simulink model "NPSS_TTECTrA_sched"  (Simulink 7.5)
settings: Solver=FixedStepDiscrete  StartTime=0.0  StopTime=20  FixedStep=0.02  RelTol=1e-3
undefined symbols (not defined in the file or in its folder): DiscIntNeverNeededParam
libraries: simulink x2
settings Model: Creator=jcsank  LastModifiedBy=jcsank

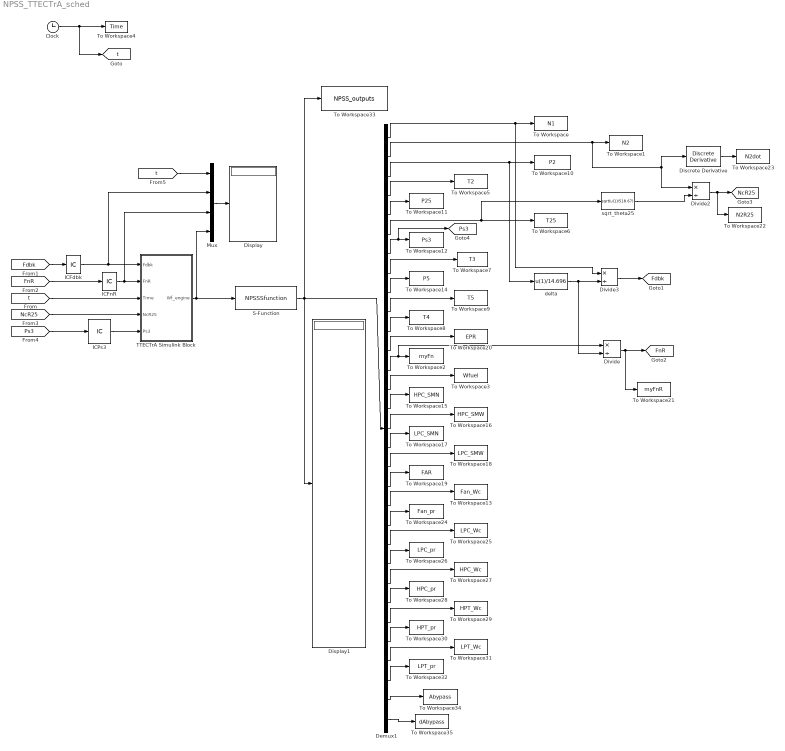
== system NPSS_TTECTrA_sched ==
  Clock : Clock
      settings: Decimation=10
  Demux1 : Demux  Outputs=31
  Discrete Derivative : simulink/Discrete/Discrete Derivative  SystemSampleTime=-1  gainval=1.0  ICPrevScaledInput=0.0  OutMin=[]  OutMax=[]  OutDataType=fixdt(1, 16)  OutScaling=2^-10  DoSatur=off
  Display : Display
  Display1 : Display
  Divide : Product  Inputs=*/
  Divide2 : Product  Inputs=*/
  Divide3 : Product  Inputs=*/
  ICFdbk : InitialCondition  Value=3325.23
  ICFnR : InitialCondition  Value=15000
  ICPs3 : InitialCondition  Value=288.259
  Mux : Mux
  S-Function : S-Function  FunctionName=NPSSSfunction  Parameters='150_PAX_Sfunction.config'  EnableBusSupport=off
  TTECTrA Simulink Block : Subsystem
  To Workspace : ToWorkspace  VariableName=N1  SampleTime=-1  SaveFormat=Array
  To Workspace1 : ToWorkspace  VariableName=N2  SampleTime=-1  SaveFormat=Array
  To Workspace10 : ToWorkspace  VariableName=P2  SampleTime=-1  SaveFormat=Array
  To Workspace11 : ToWorkspace  VariableName=P25  SampleTime=-1  SaveFormat=Array
  To Workspace12 : ToWorkspace  VariableName=Ps3  SampleTime=-1  SaveFormat=Array
  To Workspace13 : ToWorkspace  VariableName=Fan_Wc  SampleTime=-1  SaveFormat=Array
  To Workspace14 : ToWorkspace  VariableName=P5  SampleTime=-1  SaveFormat=Array
  To Workspace15 : ToWorkspace  VariableName=HPC_SMN  SampleTime=-1  SaveFormat=Array
  To Workspace16 : ToWorkspace  VariableName=HPC_SMW  SampleTime=-1  SaveFormat=Array
  To Workspace17 : ToWorkspace  VariableName=LPC_SMN  SampleTime=-1  SaveFormat=Array
  To Workspace18 : ToWorkspace  VariableName=LPC_SMW  SampleTime=-1  SaveFormat=Array
  To Workspace19 : ToWorkspace  VariableName=FAR  SampleTime=-1  SaveFormat=Array
  To Workspace2 : ToWorkspace  VariableName=myFn  SampleTime=-1  SaveFormat=Array
  To Workspace20 : ToWorkspace  VariableName=EPR  SampleTime=-1  SaveFormat=Array
  To Workspace21 : ToWorkspace  VariableName=myFnR  SampleTime=-1  SaveFormat=Array
  To Workspace22 : ToWorkspace  VariableName=N2R25  SampleTime=-1  SaveFormat=Array
  To Workspace23 : ToWorkspace  VariableName=N2dot  SampleTime=-1  SaveFormat=Array
  To Workspace24 : ToWorkspace  VariableName=Fan_pr  SampleTime=-1  SaveFormat=Array
  To Workspace25 : ToWorkspace  VariableName=LPC_Wc  SampleTime=-1  SaveFormat=Array
  To Workspace26 : ToWorkspace  VariableName=LPC_pr  SampleTime=-1  SaveFormat=Array
  To Workspace27 : ToWorkspace  VariableName=HPC_Wc  SampleTime=-1  SaveFormat=Array
  To Workspace28 : ToWorkspace  VariableName=HPC_pr  SampleTime=-1  SaveFormat=Array
  To Workspace29 : ToWorkspace  VariableName=HPT_Wc  SampleTime=-1  SaveFormat=Array
  To Workspace3 : ToWorkspace  VariableName=Wfuel  SampleTime=-1  SaveFormat=Array
  To Workspace30 : ToWorkspace  VariableName=HPT_pr  SampleTime=-1  SaveFormat=Array
  To Workspace31 : ToWorkspace  VariableName=LPT_Wc  SampleTime=-1  SaveFormat=Array
  To Workspace32 : ToWorkspace  VariableName=LPT_pr  SampleTime=-1  SaveFormat=Array
  To Workspace33 : ToWorkspace  VariableName=NPSS_outputs  SampleTime=-1  SaveFormat=Array
  To Workspace34 : ToWorkspace  VariableName=Abypass  SampleTime=-1  SaveFormat=Array
  To Workspace35 : ToWorkspace  VariableName=dAbypass  SampleTime=-1  SaveFormat=Array
  To Workspace4 : ToWorkspace  VariableName=Time  SampleTime=-1  SaveFormat=Array
  To Workspace5 : ToWorkspace  VariableName=T2  SampleTime=-1  SaveFormat=Array
  To Workspace6 : ToWorkspace  VariableName=T25  SampleTime=-1  SaveFormat=Array
  To Workspace7 : ToWorkspace  VariableName=T3  SampleTime=-1  SaveFormat=Array
  To Workspace8 : ToWorkspace  VariableName=T4  SampleTime=-1  SaveFormat=Array
  To Workspace9 : ToWorkspace  VariableName=T5  SampleTime=-1  SaveFormat=Array
  delta : Fcn  Expr=u(1)/14.696
  sqrt_theta25 : Fcn  Expr=sqrt(u(1)/518.67)
  tag scope: Fdbk=global, FnR=global, NcR25=global, Ps3=global, t=global
  wires:
  S-Function/1 -> Demux1/1, Display1/1, To Workspace33/1
  Clock/1 -> [t], To Workspace4/1
  TTECTrA Simulink Block/1(Wf_engine) -> Mux/4, S-Function/1
  [t] -> TTECTrA Simulink Block/3(Time)
  [Fdbk] -> ICFdbk/1
  [FnR] -> ICFnR/1
  [NcR25] -> TTECTrA Simulink Block/4(NcR25)
  Divide/1 -> [FnR], To Workspace21/1
  Divide2/1 -> [NcR25], To Workspace22/1
  Discrete Derivative/1 -> To Workspace23/1
  [t] -> Mux/1
  Mux/1 -> Display/1
  [Ps3] -> ICPs3/1
  Demux1/1 -> To Workspace/1, Divide3/1
  Demux1/2 -> To Workspace1/1, Divide2/1, Discrete Derivative/1
  Demux1/3 -> To Workspace10/1, delta/1
  Demux1/4 -> To Workspace5/1
  Demux1/5 -> To Workspace11/1
  Demux1/6 -> To Workspace6/1, sqrt_theta25/1
  Demux1/7 -> To Workspace12/1, [Ps3]
  Demux1/8 -> To Workspace7/1
  Demux1/10 -> To Workspace9/1
  Demux1/9 -> To Workspace14/1
  Demux1/11 -> To Workspace8/1
  Demux1/12 -> To Workspace20/1
  Demux1/13 -> To Workspace2/1, Divide/1
  Demux1/14 -> To Workspace3/1
  Demux1/15 -> To Workspace15/1
  Demux1/16 -> To Workspace16/1
  Demux1/17 -> To Workspace17/1
  Demux1/18 -> To Workspace18/1
  Demux1/19 -> To Workspace19/1
  sqrt_theta25/1 -> Divide2/2
  Divide3/1 -> [Fdbk]
  ICFdbk/1 -> TTECTrA Simulink Block/1(Fdbk), Mux/2
  ICPs3/1 -> TTECTrA Simulink Block/5(Ps3)
  ICFnR/1 -> TTECTrA Simulink Block/2("FnR "), Mux/3
  delta/1 -> Divide3/2, Divide/2
  Demux1/20 -> To Workspace13/1
  Demux1/21 -> To Workspace24/1
  Demux1/22 -> To Workspace25/1
  Demux1/23 -> To Workspace26/1
  Demux1/24 -> To Workspace27/1
  Demux1/25 -> To Workspace28/1
  Demux1/26 -> To Workspace29/1
  Demux1/27 -> To Workspace30/1
  Demux1/28 -> To Workspace31/1
  Demux1/29 -> To Workspace32/1
  Demux1/30 -> To Workspace34/1
  Demux1/31 -> To Workspace35/1

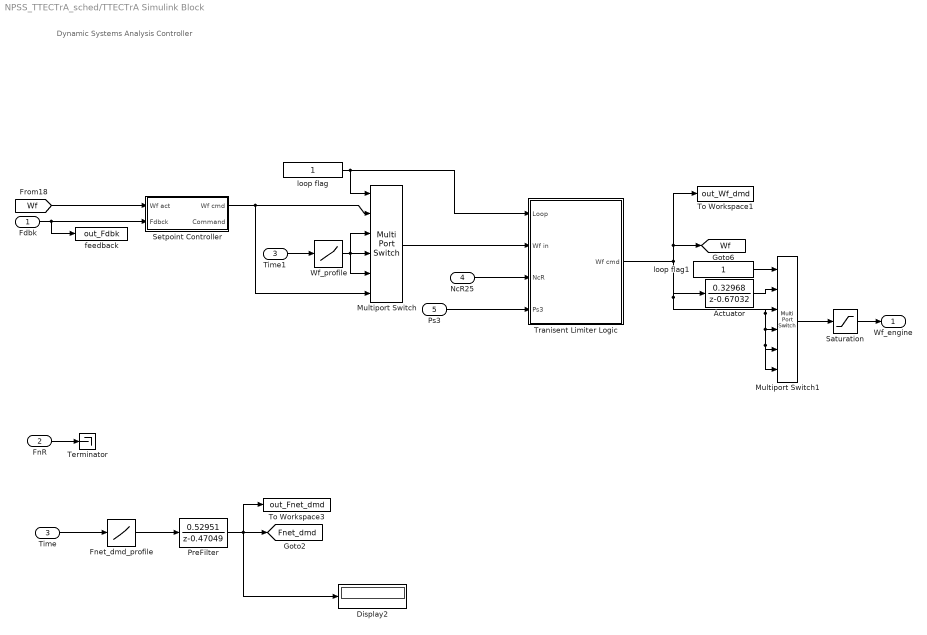
== system NPSS_TTECTrA_sched/TTECTrA Simulink Block ==
  note: Dynamic Systems Analysis Controller
  Fdbk : Inport
  "FnR " : Inport  Port=2
  Time : Inport  Port=3
  NcR25 : Inport  Port=4
  Ps3 : Inport  Port=5
  Actuator : DiscreteTransferFcn  Numerator=[0.32968]  Denominator="[1    -0.67032]"  InitialStates=[0.8029]  SampleTime=-1
  Display2 : Display
  Fnet_dmd_profile : Lookup  InputValues="[0            20            22            34            35            40          40.5            50          50.5            60            95           100]"  Table="[15000  15000  26000  26000  15000  15000  37000  37000  15000  15000  37000  37000]"  SampleTime=0.02
  Multiport Switch : MultiPortSwitch  Inputs=5  zeroidx=off  SampleTime=0.02
  Multiport Switch1 : MultiPortSwitch  Inputs=5  zeroidx=off  SampleTime=0.02
  PreFilter : DiscreteTransferFcn  Numerator=[0.52951]  Denominator="[1    -0.47049]"  InitialStates=[15000]  SampleTime=-1
  Saturation : Saturate  UpperLimit=9999  LowerLimit=0
  Setpoint Controller : Subsystem
  Terminator : Terminator
  Time1 : InportShadow  Port=3
  To Workspace1 : ToWorkspace  VariableName=out_Wf_dmd  SampleTime=-1  SaveFormat=Array
  To Workspace3 : ToWorkspace  VariableName=out_Fnet_dmd  SampleTime=-1  SaveFormat=Array
  Tranisent Limiter Logic : Subsystem
  Wf_profile : Lookup  InputValues="[0            20            22            34            35            40          40.5            50          50.5            60            95           100]"  Table="[0.5         0.5         0.5         0.5         0.5         0.5         0.5         0.5         0.5         0.5         0.5         0.5]"  SampleTime=0.02
  feedback : ToWorkspace  VariableName=out_Fdbk  SampleTime=-1  SaveFormat=Array
  loop flag : Constant
  loop flag1 : Constant
  Wf_engine : Outport
  tag scope: Fnet_dmd=global, Wf=global
  wires:
  [Wf] -> Setpoint Controller/1(Wf act)
  Fdbk/1 -> feedback/1, Setpoint Controller/2(Fdbck)
  Time/1 -> Fnet_dmd_profile/1
  NcR25/1 -> Tranisent Limiter Logic/3(NcR)
  Fnet_dmd_profile/1 -> PreFilter/1
  PreFilter/1 -> [Fnet_dmd], To Workspace3/1, Display2/1
  Saturation/1 -> Wf_engine/1
  Multiport Switch1/1 -> Saturation/1
  loop flag1/1 -> Multiport Switch1/1
  Ps3/1 -> Tranisent Limiter Logic/4(Ps3)
  Time1/1 -> Wf_profile/1
  loop flag/1 -> Tranisent Limiter Logic/1(Loop), Multiport Switch/1
  Multiport Switch/1 -> Tranisent Limiter Logic/2(Wf in)
  Wf_profile/1 -> Multiport Switch/4, Multiport Switch/3, Multiport Switch/5
  Setpoint Controller/1(Wf cmd) -> Multiport Switch/2, Multiport Switch/6
  "FnR "/1 -> Terminator/1
  Actuator/1 -> Multiport Switch1/2
  Tranisent Limiter Logic/1(Wf cmd) -> [Wf], To Workspace1/1, Actuator/1, Multiport Switch1/3, Multiport Switch1/4, Multiport Switch1/5, Multiport Switch1/6

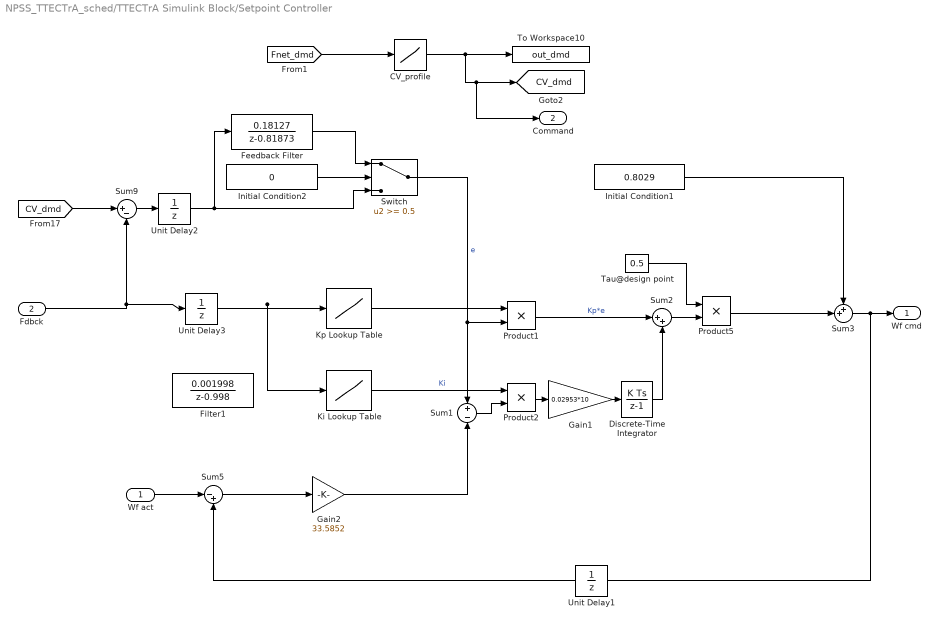
== system NPSS_TTECTrA_sched/TTECTrA Simulink Block/Setpoint Controller ==
  Wf act : Inport
  Fdbck : Inport  Port=2
  CV_profile : Lookup  InputValues="[15000  16100  17200  18300  19400  20500  21600  22700  23800  24900  26000  27100  28200  29300  30400  31500  32600  33700  34800  35900  37000]"  Table="[3325.23        3427.94        3530.34         3632.4        3727.55         3814.4        3903.37        3990.93        4076.84        4162.24        4245.48        4324.93        4403.74        4482.08        4554.24           4626        4697.19        4767.81        4837.69        4908.05        4978.43]"  LookUpMeth=Interpolation-Use End Values  SampleTime=0.02
  Discrete-Time Integrator : DiscreteIntegrator  SampleTime=-1  ICPrevOutput=DiscIntNeverNeededParam  ICPrevScaledInput=DiscIntNeverNeededParam
  Feedback Filter : DiscreteTransferFcn  Numerator=[0.18127]  Denominator="[1    -0.81873]"  SampleTime=0.02
  Filter1 : DiscreteTransferFcn  Numerator=[0.001998]  Denominator="[1      -0.998]"  SampleTime=0.02
  Gain1 : Gain  Gain=0.02953*10
  Gain2 : Gain  Gain=33.5852
  Initial Condition1 : Constant  Value=0.8029
  Initial Condition2 : Constant  Value=0
  Ki Lookup Table : Lookup_n-D  NumberOfTableDimensions=1  BreakpointsForDimension1="[3325.23        3427.94        3530.35        3632.41        3727.55         3814.4        3903.37        3990.93        4076.84        4162.24        4245.48        4324.93        4403.73        4482.08        4554.24           4626        4697.19        4767.81        4837.69        4908.05        4978.43]"  Table="[0.015051    0.015444    0.015341    0.017065    0.020046    0.020556    0.020946    0.022037    0.022631    0.023103    0.024251     0.02523    0.026308    0.028729    0.030476    0.030781    0.032445    0.033214    0.032185    0.032086    0.034071]"  SampleTime=0.02  RndMeth=Simplest  InputSameDT=on
  Kp Lookup Table : Lookup_n-D  NumberOfTableDimensions=1  BreakpointsForDimension1="[3325.23        3427.94        3530.35        3632.41        3727.55         3814.4        3903.37        3990.93        4076.84        4162.24        4245.48        4324.93        4403.73        4482.08        4554.24           4626        4697.19        4767.81        4837.69        4908.05        4978.43]"  Table="[0.0033942   0.0034271   0.0034167   0.0034139   0.0033724   0.0034011   0.0034128   0.0034016   0.0034168   0.0034462   0.0034167   0.0034099   0.0033799   0.0034958   0.0034346   0.0034205   0.0035406    0.003412   0.0037437   0.0037018   0.0038138]"  SampleTime=0.02  RndMeth=Simplest  InputSameDT=on
  Product1 : Product  SampleTime=0.02  RndMeth=Zero
  Product2 : Product  RndMeth=Zero
  Product5 : Product  SampleTime=0.02  RndMeth=Zero
  Sum1 : Sum  Inputs=+|-
  Sum2 : Sum  Inputs=|++  SampleTime=0.02
  Sum3 : Sum  Inputs=++|  SampleTime=0.02
  Sum5 : Sum  Inputs=|-+
  Sum9 : Sum  Inputs=|+-  SampleTime=0.02
  Switch : Switch  Threshold=0.5  SampleTime=0.02
  Tau@design point : Constant  Value=0.5
  To Workspace10 : ToWorkspace  VariableName=out_dmd  SampleTime=-1  SaveFormat=Array
  Unit Delay1 : UnitDelay  SampleTime=-1
  Unit Delay2 : UnitDelay  SampleTime=-1
  Unit Delay3 : UnitDelay  SampleTime=-1
  Wf cmd : Outport
  Command : Outport  Port=2
  tag scope: CV_dmd=global
  wires:
  Tau@design point/1 -> Product5/1
  Product1/1 -> Sum2/1  "Kp*e"
  Product2/1 -> Gain1/1
  Sum9/1 -> Unit Delay2/1
  [CV_dmd] -> Sum9/1
  Wf act/1 -> Sum5/1
  Sum5/1 -> Gain2/1
  Switch/1 -> Product1/2, Sum1/1  "e"
  Sum1/1 -> Product2/2
  Sum2/1 -> Product5/2
  Gain2/1 -> Sum1/2
  Sum3/1 -> Wf cmd/1, Unit Delay1/1
  Initial Condition1/1 -> Sum3/1
  Product5/1 -> Sum3/2
  Gain1/1 -> Discrete-Time Integrator/1
  Discrete-Time Integrator/1 -> Sum2/2
  Ki Lookup Table/1 -> Product2/1  "Ki"
  Fdbck/1 -> Sum9/2, Unit Delay3/1
  CV_profile/1 -> To Workspace10/1, [CV_dmd], Command/1
  [Fnet_dmd] -> CV_profile/1
  Kp Lookup Table/1 -> Product1/1
  Initial Condition2/1 -> Switch/2
  Feedback Filter/1 -> Switch/1
  Unit Delay1/1 -> Sum5/2
  Unit Delay2/1 -> Switch/3, Feedback Filter/1
  Unit Delay3/1 -> Kp Lookup Table/1, Ki Lookup Table/1

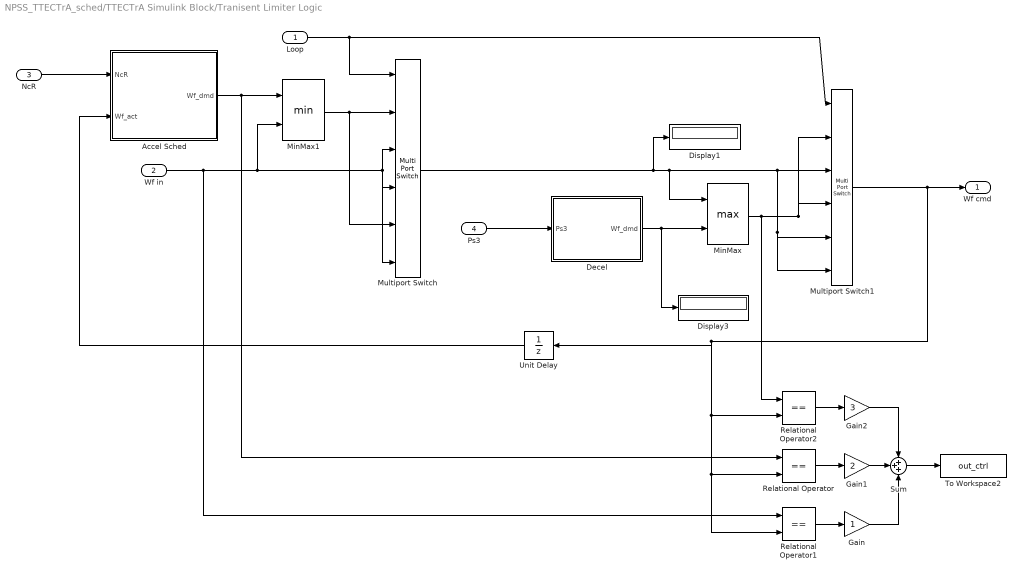
== system NPSS_TTECTrA_sched/TTECTrA Simulink Block/Tranisent Limiter Logic ==
  Loop : Inport
  Wf in : Inport  Port=2
  NcR : Inport  Port=3
  Ps3 : Inport  Port=4
  Accel Sched : Subsystem
  Decel : Subsystem
  Display1 : Display
  Display3 : Display
  Gain : Gain  ParameterDataType=fixdt(1, 16)  ParameterScaling=2^0  OutDataType=fixdt(1, 16)  OutScaling=2^0
  Gain1 : Gain  Gain=2  ParameterDataType=fixdt(1, 16)  ParameterScaling=2^0  OutDataType=fixdt(1, 16)  OutScaling=2^0
  Gain2 : Gain  Gain=3  ParameterDataType=fixdt(1, 16)  ParameterScaling=2^0  OutDataType=fixdt(1, 16)  OutScaling=2^0
  MinMax : MinMax  Function=max  Inputs=2  SampleTime=0.02
  MinMax1 : MinMax  Inputs=2  SampleTime=0.02
  Multiport Switch : MultiPortSwitch  Inputs=5  zeroidx=off  SampleTime=0.02
  Multiport Switch1 : MultiPortSwitch  Inputs=5  zeroidx=off  SampleTime=0.02
  Relational Operator : RelationalOperator  Operator===  LogicOutDataTypeMode=boolean  LogicDataType=fixdt(0, 8)  OutDataTypeStr=boolean
  Relational Operator1 : RelationalOperator  Operator===  LogicOutDataTypeMode=boolean  LogicDataType=fixdt(0, 8)  OutDataTypeStr=boolean
  Relational Operator2 : RelationalOperator  Operator===  LogicOutDataTypeMode=boolean  LogicDataType=fixdt(0, 8)  OutDataTypeStr=boolean
  Sum : Sum  Inputs=+++  OutDataType=fixdt(1, 16)  OutScaling=2^0
  To Workspace2 : ToWorkspace  VariableName=out_ctrl  SampleTime=-1  SaveFormat=Array
  Unit Delay : UnitDelay  SampleTime=-1
  Wf cmd : Outport
  wires:
  NcR/1 -> Accel Sched/1(NcR)
  Unit Delay/1 -> Accel Sched/2(Wf_act)
  Loop/1 -> Multiport Switch/1, Multiport Switch1/1
  Accel Sched/1(Wf_dmd) -> MinMax1/1, Relational Operator/1
  Wf in/1 -> Multiport Switch/3, Multiport Switch/6, Multiport Switch/4, MinMax1/2, Relational Operator1/1
  Ps3/1 -> Decel/1(Ps3)
  Multiport Switch1/1 -> Wf cmd/1, Unit Delay/1, Relational Operator2/2, Relational Operator1/2, Relational Operator/2
  MinMax/1 -> Multiport Switch1/4, Multiport Switch1/2, Relational Operator2/1
  Multiport Switch/1 -> MinMax/1, Multiport Switch1/3, Multiport Switch1/5, Multiport Switch1/6, Display1/1
  Decel/1(Wf_dmd) -> MinMax/2, Display3/1
  MinMax1/1 -> Multiport Switch/2, Multiport Switch/5
  Relational Operator2/1 -> Gain2/1
  Relational Operator/1 -> Gain1/1
  Relational Operator1/1 -> Gain/1
  Gain2/1 -> Sum/1
  Gain1/1 -> Sum/2
  Gain/1 -> Sum/3
  Sum/1 -> To Workspace2/1

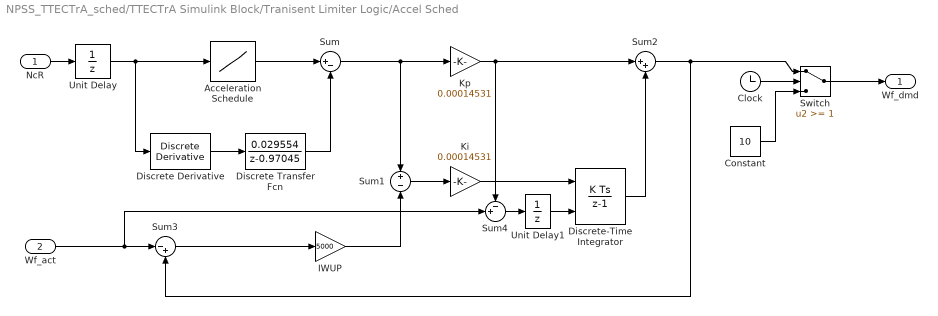
== system NPSS_TTECTrA_sched/TTECTrA Simulink Block/Tranisent Limiter Logic/Accel Sched ==
  NcR : Inport
  Wf_act : Inport  Port=2
  Acceleration Schedule : Lookup  InputValues="[11330  11371  11412  11453  11494  11535  11576  11617  11658  11699  11740  11781  11822  11863  11904  11945  11986  12027  12068  12109  12150  12191  12232  12273  12314  12355  12396  12437  12478  12519  12560  12601  12642  12683  12724  12765  12806  12847  12888  12929  12970]"  Table="[826.80549      826.80549      826.80549      826.80549      826.80549      826.80549      826.80549      826.80549      826.80549      826.80549      826.80549      826.80549      826.80549      826.80549      826.80549       2169.861      4472.7176      5790.6525      6685.5108      7356.4809      7889.4598      8320.7829      8651.7771      8926.4633      9163.2695      9366.3519      9514.0686      9602.0353      9629.1247      9600.4931      9532.9363      9449.8108        9338.03      9159.9036      826.80549      826.80549      826.80549      826.80549      826.80549      826.80549      826.80549]"  SampleTime=0.02
  Clock : Clock
      settings: Decimation=10
  Constant : Constant  Value=10  OutDataType=fixdt(1, 16)  OutScaling=2^0
  Discrete Derivative : simulink/Discrete/Discrete Derivative  SystemSampleTime=-1  gainval=1.0  ICPrevScaledInput=0  OutMin=[]  OutMax=[]  OutDataType=fixdt(1, 16)  OutScaling=2^-10  DoSatur=off
  Discrete Transfer Fcn : DiscreteTransferFcn  Numerator=[0.029554]  Denominator="[1    -0.97045]"  SampleTime=0.02
  Discrete-Time Integrator : DiscreteIntegrator  InitialConditionSource=external  SampleTime=0.02  ICPrevOutput=DiscIntNeverNeededParam  ICPrevScaledInput=DiscIntNeverNeededParam
  IWUP : Gain  Gain=5000
  Ki : Gain  Gain=0.00014531
  Kp : Gain  Gain=0.00014531  SampleTime=0.02
  Sum : Sum  Inputs=|+-  SampleTime=0.02
  Sum1 : Sum  Inputs=+|-
  Sum2 : Sum  Inputs=|++  SampleTime=0.02
  Sum3 : Sum  Inputs=|-+
  Sum4 : Sum  Inputs=-+|  SampleTime=0.02
  Switch : Switch  Threshold=1  OutDataType=fixdt(1, 16)  OutScaling=2^0
  Unit Delay : UnitDelay  SampleTime=-1
  Unit Delay1 : UnitDelay  SampleTime=-1
  Wf_dmd : Outport
  wires:
  NcR/1 -> Unit Delay/1
  Discrete Derivative/1 -> Discrete Transfer Fcn/1
  Acceleration Schedule/1 -> Sum/1
  Discrete Transfer Fcn/1 -> Sum/2
  Sum/1 -> Sum1/1, Kp/1
  Sum1/1 -> Ki/1
  Kp/1 -> Sum4/1, Sum2/1
  Sum2/1 -> Sum3/2, Switch/1
  Ki/1 -> Discrete-Time Integrator/1
  Discrete-Time Integrator/1 -> Sum2/2
  IWUP/1 -> Sum1/2
  Sum3/1 -> IWUP/1
  Wf_act/1 -> Sum4/2, Sum3/1
  Sum4/1 -> Unit Delay1/1
  Unit Delay/1 -> Discrete Derivative/1, Acceleration Schedule/1
  Unit Delay1/1 -> Discrete-Time Integrator/2
  Clock/1 -> Switch/2
  Constant/1 -> Switch/3
  Switch/1 -> Wf_dmd/1

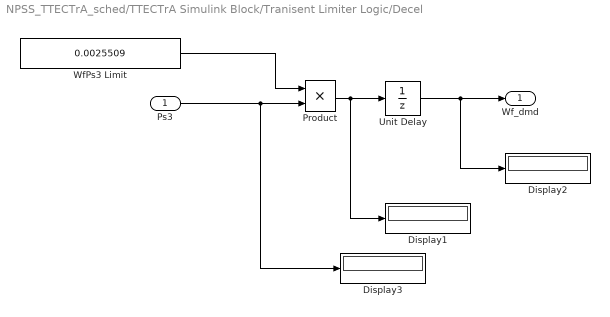
== system NPSS_TTECTrA_sched/TTECTrA Simulink Block/Tranisent Limiter Logic/Decel ==
  Ps3 : Inport
  Display1 : Display
  Display2 : Display
  Display3 : Display
  Product : Product  RndMeth=Zero
  Unit Delay : UnitDelay  X0=0.8029  SampleTime=-1
  WfPs3 Limit : Constant  Value=0.0025509
  Wf_dmd : Outport
  wires:
  Ps3/1 -> Product/2, Display3/1
  WfPs3 Limit/1 -> Product/1
  Product/1 -> Unit Delay/1, Display1/1
  Unit Delay/1 -> Wf_dmd/1, Display2/1
